simulink model "Test_THETA"  (R2019a)
settings: Solver=VariableStepAuto  StartTime=0.0  StopTime=40  RelTol=1e-3
values from neighbouring files (symbols this model uses):
  theta_x = pomocni    [Preuredi.m]
libraries: simulink x1
settings Model: Creator=branko  LastModifiedBy=branko

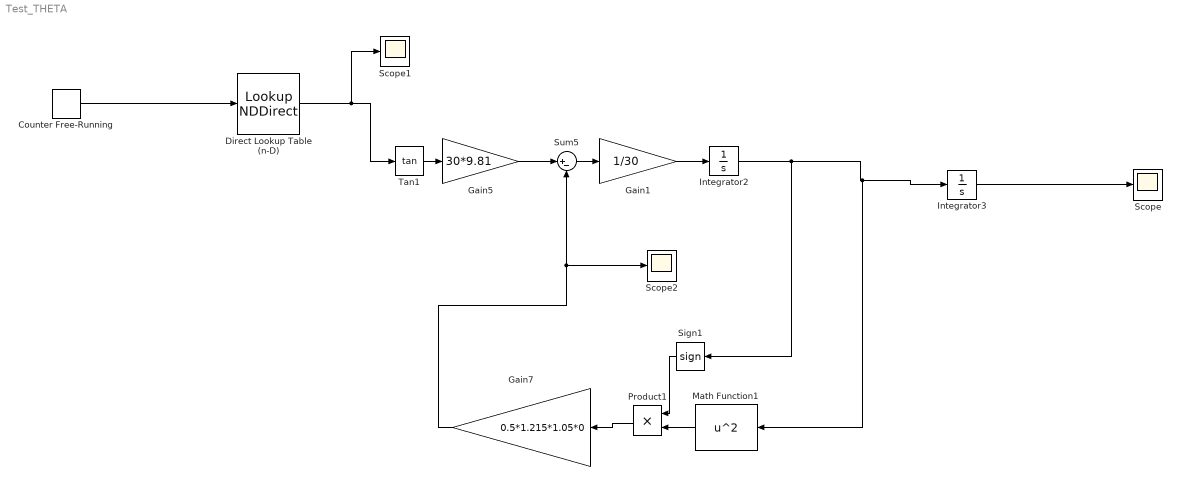
== system Test_THETA ==
  Counter Free-Running : simulink/Sources/Counter Free-Running  NumBits=32  tsamp=0.001
  Direct Lookup Table (n-D) : LookupNDDirect  NumberOfTableDimensions=1  Table=theta_x
  Gain1 : Gain  Gain=1/30
  Gain5 : Gain  Gain=30*9.81
  Gain7 : Gain  Gain=0.5*1.215*1.05*0
  Integrator2 : Integrator
  Integrator3 : Integrator
  Math Function1 : Math  Operator=square  SaturateOnIntegerOverflow=on
  Product1 : Product
  Scope : Scope
  Scope1 : Scope
  Scope2 : Scope
  Sign1 : Signum
  Sum5 : Sum  Inputs=|+-
  Tan1 : Trigonometry  Operator=tan
  wires:
  Counter Free-Running/1 -> Direct Lookup Table (n-D)/1
  ? -> ?
  Sign1/1 -> Product1/1
  Math Function1/1 -> Product1/2
  Gain7/1 -> Scope2/1, Sum5/2
  Gain5/1 -> Sum5/1
  ? -> ?
  Direct Lookup Table (n-D)/1 -> Scope1/1, Tan1/1
  Integrator2/1 -> Sign1/1, Math Function1/1, Integrator3/1
  Product1/1 -> Gain7/1
  Tan1/1 -> Gain5/1
  Gain1/1 -> Integrator2/1
  Sum5/1 -> Gain1/1
  Integrator3/1 -> Scope/1
